simulink model "DCFastChargerr"  (R2026a)
settings: Solver=ode23t  StopTime=simulation.simTime  MaxStep=1/(100*inverter.SwitchFrequency)  AbsTol=1e-3
PreLoadFcn:
  | run('params_all_evs.mlx');
InitFcn:
  | val = get_param([bdroot '/Vehicle Models'], 'Value');
  | vehicleSelect = str2double(val);
  | disp(['--- Active Vehicle Index Loaded: ', num2str(vehicleSelect), ' ---']);
  | run('params_all_evs.m');
values from neighbouring files (symbols this model uses):
  EVMaximumCurrentLimit = battery.maxPackChargeCurrent    [params_all_evs.m]
  EVMaximumVoltageLimit = battery.cellsInSeries * battery.maxCellVoltage    [params_all_evs.m]
  EVSEMaximumCurrentLimit = rectifier.DCCurrent    [params_all_evs.m]
  EVSEMaximumVoltageLimit = rectifier.DCVoltage * transformer.windingFactor    [params_all_evs.m]
undefined symbols (not defined in the file or in its folder): battery, f, inverter, rectifier
libraries: nesl_utility x34, fl_lib x22, ee_lib x14, instrumentlib x3, eePwmGenerator x2, eeTransforms x2, batteryecm_lib x1, eeSinusoidalMeasurement x1, slpidlib x1, eePwmGeneratorThreeLevel x1, eePwmGeneratorTwoLevel x1, simulink_extras x1
(part 3 of 3)

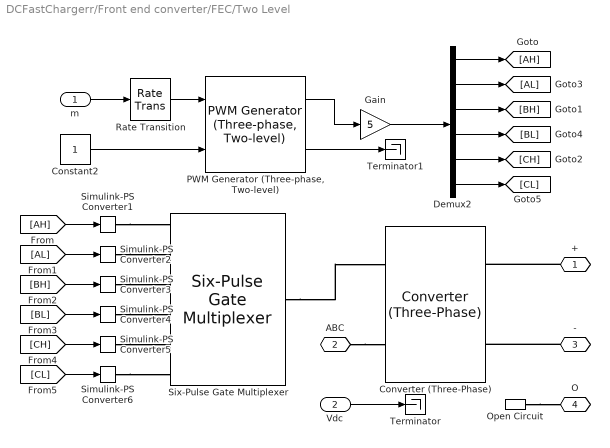
== system DCFastChargerr/Front end converter/FEC/Two Level ==
  m : Inport
  Vdc : Inport  Port=2
  Constant2 : Constant
  Converter (Three-Phase) : ee_lib/Semiconductors & Converters/Converters/Converter (Three-Phase)  port_option=ee.enum.threePhasePort.composite  fidelity_option=ee.enum.converters.fidelity.detailed  device_type=ee.enum.converters.switchingdevice.ideal  showThermalPort=false  K=0  Vth=0.5 V  Vgt=1 V  Vgt_off=-1 V  Ih=1 A  Vf=0.8 V  Ron=0.001 Ohm  Rds=0.001 Ohm  Goff=1e-6 1/Ohm  Eon_scalar=22.86e-3 J  Eoff_scalar=17.14e-3 J  Eoff_natural_commutation=10e-3 J  Voff=300 V  Iout_scalar=600 A  onCurrentMeasDelay=0 s  useCurrentFromPreviousCycle=false  useVoltageFromPreviousCycle=false  diode_param=ee.enum.converters.protectiondiode.nodynamics  diode_Vf=0.06 V  diode_Ron=0.001 Ohm  diode_Goff=1e-5 1/Ohm  diode_C=50 nF  diode_iRM=-235 A  diode_iF=300 A  diode_idot=-50 A/us  diode_trr_param=ee.enum.converters.diodetrr.trr_factor  diode_trr_factor=3  diode_trr=15 us  diode_Qrr=1500 s*uA  diode_rec_loss_model=ee.enum.diode.reverseRecoveryModel.fixed  diode_ErecVal=0 J  diode_scaleWithIandV=false  diode_ErecMat=zeros(2, 3) J  diode_TjrecVec=[298.15, 398.15] K  diode_IfrecVec=[.1, 1, 10] A  diode_IrecVal=10 A  diode_VrecVal=10 V  diode_tFilter=1 / 1000 / 100 s  thermal_network_parameterization=ee.enum.thermalNetworkTopology.external  Rth=[.08, .5] K/W  Rth_Cauer=[.08, .1, .5] K/W  Rth_Foster=[.08, .14, .22, .16] K/W  thermal_mass_parameterization=ee.enum.thermalNetwork.timeconstant  thermal_mass=[.01, .5] J/K  thermal_mass_Cauer=[.01, .1, .5] J/K  thermal_mass_Foster=[.001, .005, .05, .5] J/K  thermal_time_constant=[.001, .2] s  thermal_time_constant_Cauer=[.001, .1, .2] s  thermal_time_constant_Foster=[7e-05, .0007, .01, .08] s  thermal_mass_initial_temperatures=[25, 25] degC  thermal_mass_initial_temperatures_Cauer=[25, 25, 25] degC  junction_thermal_mass=0.01 J/K  Tvec_initial_Foster=[25, 25, 25, 25] degC  snubber_type=ee.enum.converters.snubber.exclude  Cs=1e-7 F  Rs=0.1 Ohm  Vce_loss=[0, 150, 300] V
  Demux2 : Demux  Outputs=6
  Gain : Gain  Gain=5
  Open Circuit : fl_lib/Electrical/Electrical Elements/Open Circuit  v_specify=off  v_priority=None  v=0 V  v_nominal_specify=off  v_nominal_value=1  v_nominal_unit=V
  "PWM Generator (Three-phase, Two-level)" : eePwmGeneratorTwoLevel/PWM Generator (Three-phase, Two-level)  PWMMode=Continuous PWM (CPWM)  CPWMMode=SVM: space vector modulation  DPWMMode=60 DPWM: 60 degree discontinuous PWM  fsw=rectifier.SwitchFrequency  Ts=rectifier.VoltageSensorT
  Rate Transition : RateTransition  OutPortSampleTime=rectifier.VoltageSensorT
  Simulink-PS Converter{1..6} (6 alike) : nesl_utility/Simulink-PS Converter  PhysicalDomain=network_engine_domain  SubClassName=ps_input  LeftPortType=input  RightPortType=output  PseudoPeriodic=off  Frequencies=[]  NoiseDistribution=none  NoiseParameters=[]  Unit=1  AffineConversion=off  FilteringAndDerivatives=provide  SimscapeFilterOrder=1  InputFilterTimeConstant=0.001  UdotUserProvided=0
  Six-Pulse Gate Multiplexer : ee_lib/Semiconductors & Converters/Converters/Six-Pulse Gate Multiplexer  port_option=ee.enum.controlport.ps
  Terminator : Terminator
  Terminator1 : Terminator
  + : PMIOPort  Side=Right
  ABC : PMIOPort  Port=2  Side=Left
  - : PMIOPort  Port=3  Side=Right
  O : PMIOPort  Port=4  Side=Right
  wires:
  [AH] -> Simulink-PS Converter1/1
  [CL] -> Simulink-PS Converter6/1
  [AL] -> Simulink-PS Converter2/1
  [BL] -> Simulink-PS Converter4/1
  [CH] -> Simulink-PS Converter5/1
  [BH] -> Simulink-PS Converter3/1
  Gain/1 -> Demux2/1
  Rate Transition/1 -> "PWM Generator (Three-phase, Two-level)"/1
  Demux2/2 -> [AL]
  Demux2/1 -> [AH]
  Demux2/5 -> [CH]
  Demux2/3 -> [BH]
  "PWM Generator (Three-phase, Two-level)"/1 -> Gain/1
  Demux2/4 -> [BL]
  Demux2/6 -> [CL]
  Constant2/1 -> "PWM Generator (Three-phase, Two-level)"/2
  m/1 -> Rate Transition/1
  Vdc/1 -> Terminator/1
  "PWM Generator (Three-phase, Two-level)"/2 -> Terminator1/1
  connections:
  ABC/RConn1 -- Converter (Three-Phase)/LConn2
  Simulink-PS Converter1/RConn1 -- Six-Pulse Gate Multiplexer/LConn1
  Simulink-PS Converter2/RConn1 -- Six-Pulse Gate Multiplexer/LConn2
  Simulink-PS Converter3/RConn1 -- Six-Pulse Gate Multiplexer/LConn3
  Simulink-PS Converter4/RConn1 -- Six-Pulse Gate Multiplexer/LConn4
  Simulink-PS Converter5/RConn1 -- Six-Pulse Gate Multiplexer/LConn5
  Simulink-PS Converter6/RConn1 -- Six-Pulse Gate Multiplexer/LConn6
  Six-Pulse Gate Multiplexer/RConn1 -- Converter (Three-Phase)/LConn1
  +/RConn1 -- Converter (Three-Phase)/RConn1
  -/RConn1 -- Converter (Three-Phase)/RConn2
  Open Circuit/LConn1 -- O/RConn1

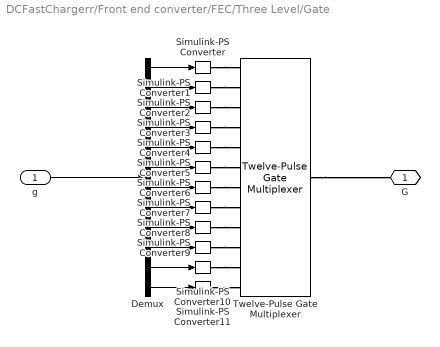
== system DCFastChargerr/Front end converter/FEC/Three Level/Gate ==
  g : Inport
  Demux : Demux  Outputs=12
  Simulink-PS Converter{,1..11} (12 alike) : nesl_utility/Simulink-PS Converter  PhysicalDomain=network_engine_domain  SubClassName=ps_input  LeftPortType=input  RightPortType=output  PseudoPeriodic=off  Frequencies=[]  NoiseDistribution=none  NoiseParameters=[]  Unit=1  AffineConversion=off  FilteringAndDerivatives=zero  SimscapeFilterOrder=1  InputFilterTimeConstant=0.001  UdotUserProvided=1
  Twelve-Pulse Gate Multiplexer : ee_lib/Semiconductors & Converters/Converters/Twelve-Pulse Gate Multiplexer  port_option=ee.enum.controlport.ps
  G : PMIOPort  Side=Right
  wires:
  g/1 -> Demux/1
  Demux/5 -> Simulink-PS Converter4/1
  Demux/10 -> Simulink-PS Converter9/1
  Demux/2 -> Simulink-PS Converter1/1
  Demux/9 -> Simulink-PS Converter8/1
  Demux/12 -> Simulink-PS Converter11/1
  Demux/3 -> Simulink-PS Converter2/1
  Demux/7 -> Simulink-PS Converter6/1
  Demux/6 -> Simulink-PS Converter5/1
  Demux/4 -> Simulink-PS Converter3/1
  Demux/1 -> Simulink-PS Converter/1
  Demux/11 -> Simulink-PS Converter10/1
  Demux/8 -> Simulink-PS Converter7/1
  connections:
  Simulink-PS Converter10/RConn1 -- Twelve-Pulse Gate Multiplexer/LConn11
  Simulink-PS Converter8/RConn1 -- Twelve-Pulse Gate Multiplexer/LConn9
  Simulink-PS Converter/RConn1 -- Twelve-Pulse Gate Multiplexer/LConn1
  Simulink-PS Converter11/RConn1 -- Twelve-Pulse Gate Multiplexer/LConn12
  Simulink-PS Converter3/RConn1 -- Twelve-Pulse Gate Multiplexer/LConn4
  Simulink-PS Converter2/RConn1 -- Twelve-Pulse Gate Multiplexer/LConn3
  Simulink-PS Converter4/RConn1 -- Twelve-Pulse Gate Multiplexer/LConn5
  Simulink-PS Converter1/RConn1 -- Twelve-Pulse Gate Multiplexer/LConn2
  Twelve-Pulse Gate Multiplexer/RConn1 -- G/RConn1
  Simulink-PS Converter5/RConn1 -- Twelve-Pulse Gate Multiplexer/LConn6
  Simulink-PS Converter9/RConn1 -- Twelve-Pulse Gate Multiplexer/LConn10
  Simulink-PS Converter6/RConn1 -- Twelve-Pulse Gate Multiplexer/LConn7
  Simulink-PS Converter7/RConn1 -- Twelve-Pulse Gate Multiplexer/LConn8

== system DCFastChargerr/Front end converter/FEC/Three Level/Sensing voltage Vc1 ==
  PS-Simulink Converter : nesl_utility/PS-Simulink Converter  PhysicalDomain=network_engine_domain  SubClassName=ps_output  LeftPortType=input  RightPortType=output  PseudoPeriodic=off  Frequencies=[]  VectorFormat=1-D array  Unit=1  AffineConversion=off
  Sensor dynamics : TransferFcn  Numerator=rectifier.VoltageSensorG  Denominator=[rectifier.VoltageSensorT 1]
  Vc1 : fl_lib/Electrical/Electrical Sensors/Voltage Sensor
  + : PMIOPort  Side=Left
  - : PMIOPort  Port=2  Side=Right
  Out1 : Outport
  wires:
  PS-Simulink Converter/1 -> Sensor dynamics/1
  Sensor dynamics/1 -> Out1/1
  connections:
  Vc1/RConn2 -- -/RConn1
  Vc1/LConn1 -- +/RConn1
  PS-Simulink Converter/LConn1 -- Vc1/RConn1

== system DCFastChargerr/Front end converter/FEC/Three Level/Sensing voltage Vc2 ==
  PS-Simulink Converter : nesl_utility/PS-Simulink Converter  PhysicalDomain=network_engine_domain  SubClassName=ps_output  LeftPortType=input  RightPortType=output  PseudoPeriodic=off  Frequencies=[]  VectorFormat=1-D array  Unit=1  AffineConversion=off
  Sensor dynamics : TransferFcn  Numerator=rectifier.VoltageSensorG  Denominator=[rectifier.VoltageSensorT 1]
  Vc2 : fl_lib/Electrical/Electrical Sensors/Voltage Sensor
  Conn1 : PMIOPort  Side=Left
  Conn3 : PMIOPort  Port=2  Side=Right
  Out1 : Outport
  wires:
  Sensor dynamics/1 -> Out1/1
  PS-Simulink Converter/1 -> Sensor dynamics/1
  connections:
  Vc2/RConn2 -- Conn3/RConn1
  Vc2/LConn1 -- Conn1/RConn1
  PS-Simulink Converter/LConn1 -- Vc2/RConn1

== stateflow chart DCFastChargerr/OCPP_Supervisor ==
  state AuthorizeState
    entry:
    auth_timer = 0;
    during:
    auth_timer = auth_timer + 1;
    if auth_timer < 50
    MessageCode = uint8(2);
    else
    MessageCode = uint8(0);
    end
  state StopSession
    entry:
    MessageCode = uint8(5);
    OCPP_Authorized = false;
  state BootingState
    entry: MessageCode = 1; OCPP_Authorized = false;
  state IdleState
    entry:
    MessageCode = uint8(0);
    auth_sent = false;
  state ChargingSession
    entry:
    OCPP_Authorized = true;
    telemetry_timer = 0;
    during:
    telemetry_timer = telemetry_timer + 1;
    % Start Transaction (Message 3) pulse for first 50ms
    if telemetry_timer < 50
    MessageCode = uint8(3);
    % Meter Values (Message 4) pulse for 50ms every 5 seconds (5000 ticks)
    elseif mod(telemetry_timer, 5000) < 50
    MessageCode = uint8(4);
    % Mute transmission between pulses
    else
    MessageCode = uint8(0);
    end
  (default) -> BootingState
  AuthorizeState -> StopSession [order 2] : [UDP_Status == 1 && UDP_Data(1) == 48]
  BootingState -> IdleState : after(0.01, sec)
  IdleState -> AuthorizeState : [PlugConnected == true]
  ChargingSession -> StopSession : [SOC >= 0.95]
  AuthorizeState -> ChargingSession [order 1] : [OCPP_Authorized == true || (UDP_Status == 1 && UDP_Data(1) == 49)]
  data: MessageCode output uint8 size=1; OCPP_Authorized output boolean size=1; UDP_Data input uint8 size=16; UDP_Status input uint8 size=1; PlugConnected input boolean size=1; SOC input double size=1; auth_sent local boolean size=1; telemetry_timer local double; auth_timer local

== matlab function DCFastChargerr/MATLAB Function ==
  data: MessageCode input; udp_bytes_out output; VehicleSelect input; LivePower_W input
function udp_bytes_out = format_ocpp_msg(MessageCode, VehicleSelect, LivePower_W)
    % Pre-allocate fixed-size output array for code generation safety
    udp_bytes_out = zeros(1, 40, 'uint8'); 
    
    if MessageCode == 0
        return;
    end
    
    switch VehicleSelect
        case 1
            tag = 'TAG_LEAF_01';
        case 2
            tag = 'TAG_EV6_02';
        case 3
            tag = 'TAG_TESLA_03';
        case 4
            tag = 'TAG_RIVIAN_04';
        case 5
            tag = 'TAG_BOLT_05';
        otherwise
            tag = 'UNKNOWN_TAG';
    end
    
    msg_code_char = uint8(MessageCode + 48); 
    
    if MessageCode == 2 % Authorize
        str_data = [char(msg_code_char), ',', tag];
    elseif MessageCode == 3 % StartTransaction
        str_data = [char(msg_code_char), ',', tag];
    elseif MessageCode == 4 % MeterValues (Live Telemetry)
        power_val_int = int32(round(LivePower_W));
        power_str = sprintf('%d', power_val_int);
        str_data = [char(msg_code_char), ',', power_str];
    elseif MessageCode == 5 % StopTransaction
        str_data = char(msg_code_char);
    else
        str_data = char(msg_code_char);
    end
    
    % Safely map to fixed-size buffer to prevent coder dimension mismatch errors
    len = min(length(str_data), 40);
    udp_bytes_out(1:len) = uint8(str_data(1:len));
end

== stateflow chart DCFastChargerr/EVCC_SECC_Handshake/Chart ==
  settings: sampleTime=0.001
  state CurrentDemand
    during:
    % 1. CC-CV Demand Curve (Tapering from 85% to 95% SOC)
    if SOC < 0.85
    % Bulk charge phase: request maximum allowed current
    EVTargetCurrent = EVMaximumCurrentLimit;
    else
    % Taper phase: linearly ramp down current from 85% to 95% SOC
    EVTargetCurrent = EVMaximumCurrentLimit * ((0.95 - SOC) / 0.10);
    end
    % 2. Voltage Safety Guard & ISO 15118 Dynamic Negotiation
    if isempty(Vbat) || Vbat(1) < 10.0
    Vbat_safe = 300.0;
    else
    Vbat_safe = Vbat(1);
    end
    EVMaximumPowerLimit = EVMaximumVoltageLimit * EVMaximumCurrentLimit;
    EVMaxPowerCurrent = EVMaximumPowerLimit / Vbat_safe;
    EVSEMaxPower = EVSEMaximumVoltageLimit * EVSEMaximumCurrentLimit;
    EVSEMaxPowerCurrent = EVSEMaxPower / Vbat_safe;
    % Strict scalar bounds: clamp EV target against battery limits, hardware limits, and Cloud limits
    NegotiatedCurrent = min([EVTargetCurrent, EVMaximumCurrentLimit, EVSEMaximumCurrentLimit, EVMaxPowerCurrent, EVSEMaxPowerCurrent, GridCurrentLimit]);
    % 3. Output the negotiated value directly — slew-rate limiting now handled
    % OUTSIDE this chart by a Rate Limiter block (500 A/s rising, -500 A/s falling)
    % on the CurrentReference output wire. Do NOT re-add step-based ramping here.
    CurrentReference = NegotiatedCurrent;
  state SessionSetup
    entry: CurrentReference = 0; ChargingEnable = false;
  state Authorization
    entry: CurrentReference = 0; ChargingEnable = false; OCPP_Authorized == true;
    % placeholder - will gate on OCPP Authorize.conf
  state ServiceDiscovery
    entry:
    CurrentReference = 0;
    ChargingEnable = false;
  state ChargeParameterDiscovery
    entry:
    CurrentReference = 0;
    ChargingEnable = false;
  state PowerDelivery
    entry:
    % PHYSICAL: Close Pre-Charge Relay (PCR). Main positive contactor is OPEN.
    % LOGIC: Command charger to wake up and match pack voltage at 0 Amps.
    ChargingEnable = true;
    CurrentReference = 0;
  state SessionStop
    entry:
    CurrentReference = 0;
    ChargingEnable = false;
  (default) -> SessionSetup
  SessionSetup -> Authorization
  Authorization -> ServiceDiscovery
  ServiceDiscovery -> ChargeParameterDiscovery : after(0.01,sec)
  PowerDelivery -> CurrentDemand
  CurrentDemand -> SessionStop : [SOC>=0.95]
  ChargeParameterDiscovery -> PowerDelivery
  data: CurrentReference output double; ChargingEnable output boolean; SOC input; Ibat input; TargetCurrent local; Vdc input size=1; Vbat input; EVMaximumCurrentLimit input double; EVMaximumVoltageLimit input double; EVTargetCurrent local double; NegotiatedCurrent local double; MaxPowerCurrent local double; EVMaxPowerCurrent local; EVSEMaxPower local; EVSEMaxPowerCurrent local; EVMaximumPowerLimit local double; EVSEMaximumCurrentLimit input double; EVSEMaximumVoltageLimit input; OCPP_Authorized input boolean; GridCurrentLimit input double; rate_step local; Vbat_safe local
